simulink model "sim_quadrotor"  (R2015a)
settings: Solver=ode3  StartTime=0  StopTime=inf  FixedStep=quadEDT.sampletime  MaxStep=0.1  RelTol=1e-3
InitFcn:
  | % load parameters of the default quadrotor
  | disp('Quadrotor parameters loaded by InitFcn')
  | parameters_estimationcontrol %loads mdl_quadcopter, too!
  | 
  | % change to Simulation folder if in data folder
  | cd([matlabpath '/Simulation']);
undefined symbols (not defined in the file or in its folder): controlHelperParams, Discrete, estimParams, quad, quadEDT, Time
libraries: simulink x30, ctrlSharedLib x3, vrlib x1, commnoisgen2 x1, aerolibtransform2 x1
(part 2 of 2)

== system sim_quadrotor/Drone_Compensator/Estimator/EstimatorXYPosition/EstimatorXYPosition ==
  note: Switching from orientationControl to Position control reset the current world position estimate (happens when using no markers!)
  dxy_estimin : Inport
  orient_estimin : Inport  Port=2
  controlModePosVSOrient_flagin : Inport  Port=3
  dz_estimin : Inport  Port=4
  posVIS_datin : Inport  Port=5
  usePosVIS_flagin : Inport  Port=6
  Delay : Delay  DelayLength=1  InitialCondition=0
  KalmanFilter_posxy : ctrlSharedLib/Kalman Filter  TimeDomain=Discrete-Time  UseCurrentEstimator=on  ModelSource=Individual A, B, C, D matrices  ModelSourceVariable=ss(0.95,1,1,0,1)  A=eye(2)  B=quadEDT.sampletime*eye(2)  C=eye(2)  D=0  NumberOfStates=1  NumberOfInputs=1  NumberOfOutputs=1  InitialEstimateSource=Dialog  X0=[.1 0.0]  P0=10  UseK=off  UseGH=on  NumberOfProcessNoiseInputs=1  G=estimParams.pos.kfpos.G  TimeInvariantG=on  H=estimParams.pos.kfpos.H  TimeInvariantH=on  Q=estimParams.pos.kfpos.Q  TimeInvariantQ=on  R=estimParams.pos.kfpos.R  TimeInvariantR=on  N=estimParams.pos.kfpos.N  TimeInvariantN=on  AddInputPort=on  AddEnablePort=on  OutputEstimatedY=off  OutputP=off  Ts=-1
  Mux2 : Mux  Inputs=2
  OutlierHandling : Subsystem
  SelectXY : Selector  InputPortWidth=4  Indices=[1 2]
  SelectdXY : Selector  InputPortWidth=3  Indices=[1 2]
  SimplyIntegrateVelocity : DiscreteIntegrator  ExternalReset=rising  InitialConditionSetting=State (most efficient)  SampleTime=quadEDT.sampletime  LimitOutput=on  UpperSaturationLimit=estimParams.pos.veloIntegrator_max  LowerSaturationLimit=-estimParams.pos.veloIntegrator_max
  UseIPPosSwitch : Switch  Criteria=u2 > Threshold
  trafo_BodytoWorld_trans : MATLAB Function  TreatAsAtomicUnit=on
  XY_estimout : Outport
  wires:
  orient_estimin/1 -> trafo_BodytoWorld_trans/1(orientation), OutlierHandling/1(orient_estimin)
  dxy_estimin/1 -> Mux2/1
  SimplyIntegrateVelocity/1 -> UseIPPosSwitch/3
  dz_estimin/1 -> Mux2/2
  Mux2/1 -> trafo_BodytoWorld_trans/2(vector)
  trafo_BodytoWorld_trans/1(vel_world) -> SelectdXY/1
  SelectdXY/1 -> KalmanFilter_posxy/1, SimplyIntegrateVelocity/1
  posVIS_datin/1 -> SelectXY/1, OutlierHandling/2(posVIS_datin)
  KalmanFilter_posxy/1 -> Delay/1, UseIPPosSwitch/1
  controlModePosVSOrient_flagin/1 -> SimplyIntegrateVelocity/2
  UseIPPosSwitch/1 -> XY_estimout/1
  usePosVIS_flagin/1 -> UseIPPosSwitch/2
  SelectXY/1 -> KalmanFilter_posxy/2
  OutlierHandling/1(enable_flag) -> KalmanFilter_posxy/3
  Delay/1 -> OutlierHandling/3(pos_estim)

== system sim_quadrotor/SimulatorDrone/DroneRS_Sensorsystem/IMU_Pressure/ Noise ==
  states_datin : Inport
  Add : Sum
  Bus Creator : BusCreator  Inputs='X','Y','Z','yaw','pitch','roll','dx','dy','dz','p','q','r'
  Bus to Vector : BusToVector
  Demux1 : Demux  Outputs=12
  Gaussian Noise Generator : commnoisgen2/Gaussian Noise Generator  m=0  d=quadEDT.noiseStatesSensed_std.^2  s=41  Ts=quadEDT.sampletime  frameBased=off  sampPerFrame=1  orient=off  outDataType=double
  noiseWeights : Gain  Gain=quadEDT.noiseStatesSensed_weights
  states_noisy_datout : Outport
  wires:
  Bus Creator/1 -> states_noisy_datout/1
  Gaussian Noise Generator/1 -> noiseWeights/1
  Demux1/6 -> Bus Creator/6  "roll"
  Add/1 -> Demux1/1
  Demux1/8 -> Bus Creator/8  "dy"
  Demux1/10 -> Bus Creator/10  "p"
  Demux1/12 -> Bus Creator/12  "r"
  Demux1/2 -> Bus Creator/2  "Y"
  Bus to Vector/1 -> Add/1
  Demux1/3 -> Bus Creator/3  "Z"
  Demux1/7 -> Bus Creator/7  "dx"
  Demux1/9 -> Bus Creator/9  "dz"
  Demux1/4 -> Bus Creator/4  "yaw"
  Demux1/11 -> Bus Creator/11  "q"
  states_datin/1 -> Bus to Vector/1
  Demux1/5 -> Bus Creator/5  "pitch"
  Demux1/1 -> Bus Creator/1  "X"
  noiseWeights/1 -> Add/2

== system sim_quadrotor/Drone_Compensator/Estimator/EstimatorXYPosition/EstimatorVelocity/AccelerationHandling ==
  dxy_estimin : Inport
  orient_estimin : Inport  Port=2
  sensorIMU_datin : Inport  Port=3
  Z_estimin : Inport  Port=4
  Add : Sum  Inputs=-+
  Bus Selector1 : BusSelector  OutputSignals=ddx,ddy,ddz
  Deactivate Acceleration If OF is not used due to low altitude : simulink/Logic and Bit Operations/Compare To Constant  relop=<=  const=estimParams.pos.opticalFlow_Z_max  OutDataTypeStr=boolean
  Logical Operator : Logic  Operator=OR  AllPortsSameDT=off  OutDataTypeStr=boolean
  Mux6 : Mux  Inputs=3
  Product : Product  Inputs=3
  SelectPlanarddxy : Selector  InputPortWidth=3  Indices=[1 2]
  Selector : Selector  InputPortWidth=2
  Selector1 : Selector  InputPortWidth=2  Indices=2
  do not use acc if optical flow never available (Note OF@60Hz but ZOH to 200!) : simulink/Logic and Bit Operations/Compare To Constant  relop=~=  const=0  OutDataTypeStr=boolean
  do not use acc if optical flow never available (Note OF@60Hz but ZOH to 200!)1 : simulink/Logic and Bit Operations/Compare To Constant  relop=~=  const=0  OutDataTypeStr=boolean
  gainaccinput : Gain  Gain=estimParams.pos.accelerationInput_gain
  gravity : Constant  Value=[0 0 -quad.g]
  trafo_World2Body_trans : MATLAB Function  TreatAsAtomicUnit=on
  acceleration_world : Outport
  wires:
  orient_estimin/1 -> trafo_World2Body_trans/1(orientation)
  Bus Selector1/2 -> Mux6/2  "<ddy>"
  Mux6/1 -> Add/2
  sensorIMU_datin/1 -> Bus Selector1/1
  Bus Selector1/1 -> Mux6/1  "<ddx>"
  Bus Selector1/3 -> Mux6/3  "<ddz>"
  SelectPlanarddxy/1 -> gainaccinput/1
  gainaccinput/1 -> Product/2
  gravity/1 -> trafo_World2Body_trans/2(vector)
  trafo_World2Body_trans/1(y) -> Add/1
  Add/1 -> SelectPlanarddxy/1
  Z_estimin/1 -> Deactivate Acceleration If OF is not used due to low altitude/1
  Deactivate Acceleration If OF is not used due to low altitude/1 -> Product/3
  Product/1 -> acceleration_world/1
  dxy_estimin/1 -> Selector/1, Selector1/1
  Selector/1 -> do not use acc if optical flow never available (Note OF@60Hz but ZOH to 200!)/1
  Selector1/1 -> do not use acc if optical flow never available (Note OF@60Hz but ZOH to 200!)1/1
  Logical Operator/1 -> Product/1
  do not use acc if optical flow never available (Note OF@60Hz but ZOH to 200!)/1 -> Logical Operator/1
  do not use acc if optical flow never available (Note OF@60Hz but ZOH to 200!)1/1 -> Logical Operator/2

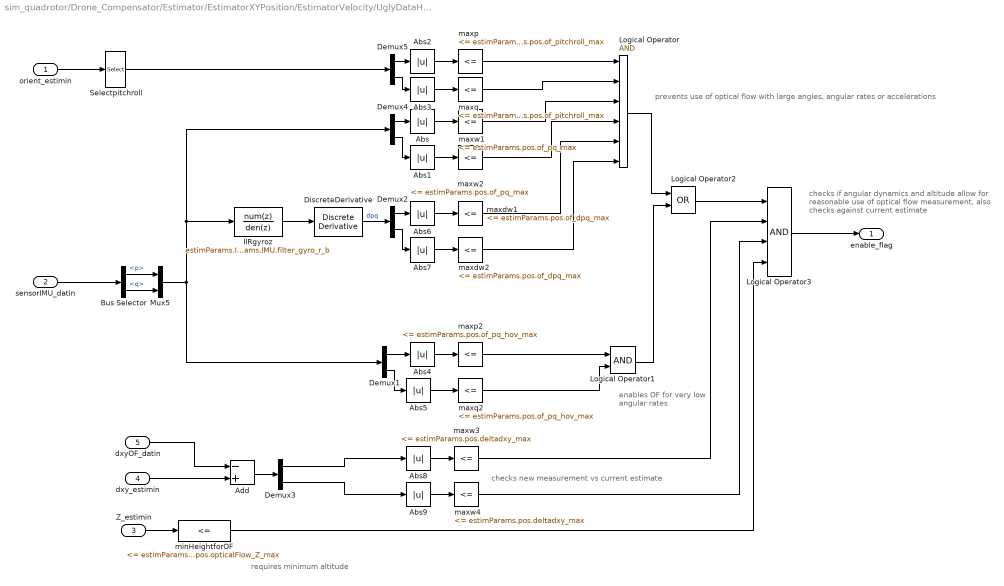
== system sim_quadrotor/Drone_Compensator/Estimator/EstimatorXYPosition/EstimatorVelocity/UglyDataHandling ==
  note: requires minimum altitude
  note: checks new measurement vs current estimate
  note: checks if angular dynamics and altitude allow for
      | reasonable use of optical flow measurement,
      | also checks against current estimate
  note: enables OF for very
      | low angular rates
  note: prevents use of optical flow with large angles, angular rates or accelerations
  orient_estimin : Inport
  sensorIMU_datin : Inport  Port=2
  Z_estimin : Inport  Port=3
  dxy_estimin : Inport  Port=4
  dxyOF_datin : Inport  Port=5
  Abs{,1..9} (10 alike) : Abs
  Add : Sum  Inputs=-+
  Bus Selector : BusSelector  OutputSignals=p,q
  Demux{1..5} (5 alike) : Demux  Outputs=2
  DiscreteDerivative : simulink/Discrete/Discrete Derivative  gainval=1.0  ICPrevScaledInput=0.0  InputProcessing=Inherited  OutMin=[]  OutMax=[]  OutDataType=fixdt(1, 16)  OutScaling=2^-10  DoSatur=off
  IIRgyroz : DiscreteFilter  Numerator=estimParams.IMU.filter_gyro_r_b  Denominator=estimParams.IMU.filter_gyro_r_b
  Logical Operator : Logic  Inputs=6  AllPortsSameDT=off  OutDataTypeStr=boolean
  Logical Operator1 : Logic  AllPortsSameDT=off  OutDataTypeStr=boolean
  Logical Operator2 : Logic  Operator=OR  AllPortsSameDT=off  OutDataTypeStr=boolean
  Logical Operator3 : Logic  Inputs=4  AllPortsSameDT=off  OutDataTypeStr=boolean
  Mux5 : Mux  Inputs=2
  Selectpitchroll : Selector  InputPortWidth=3  Indices=[2 3]
  maxdw1 : simulink/Logic and Bit Operations/Compare To Constant  relop=<=  const=estimParams.pos.of_dpq_max  OutDataTypeStr=boolean
  maxdw2 : simulink/Logic and Bit Operations/Compare To Constant  relop=<=  const=estimParams.pos.of_dpq_max  OutDataTypeStr=boolean
  maxp : simulink/Logic and Bit Operations/Compare To Constant  relop=<=  const=estimParams.pos.of_pitchroll_max  OutDataTypeStr=boolean
  maxp2 : simulink/Logic and Bit Operations/Compare To Constant  relop=<=  const=estimParams.pos.of_pq_hov_max  OutDataTypeStr=boolean
  maxq : simulink/Logic and Bit Operations/Compare To Constant  relop=<=  const=estimParams.pos.of_pitchroll_max  OutDataTypeStr=boolean
  maxq2 : simulink/Logic and Bit Operations/Compare To Constant  relop=<=  const=estimParams.pos.of_pq_hov_max  OutDataTypeStr=boolean
  maxw1 : simulink/Logic and Bit Operations/Compare To Constant  relop=<=  const=estimParams.pos.of_pq_max  OutDataTypeStr=boolean
  maxw2 : simulink/Logic and Bit Operations/Compare To Constant  relop=<=  const=estimParams.pos.of_pq_max  OutDataTypeStr=boolean
  maxw3 : simulink/Logic and Bit Operations/Compare To Constant  relop=<=  const=estimParams.pos.deltadxy_max  OutDataTypeStr=boolean
  maxw4 : simulink/Logic and Bit Operations/Compare To Constant  relop=<=  const=estimParams.pos.deltadxy_max  OutDataTypeStr=boolean
  minHeightforOF : simulink/Logic and Bit Operations/Compare To Constant  relop=<=  const=estimParams.pos.opticalFlow_Z_max  OutDataTypeStr=boolean
  enable_flag : Outport
  wires:
  maxp2/1 -> Logical Operator1/1
  Demux5/2 -> Abs3/1
  Demux5/1 -> Abs2/1
  maxq/1 -> Logical Operator/2
  maxdw2/1 -> Logical Operator/6
  maxdw1/1 -> Logical Operator/5
  orient_estimin/1 -> Selectpitchroll/1
  maxw2/1 -> Logical Operator/4
  maxp/1 -> Logical Operator/1
  Bus Selector/2 -> Mux5/2  "<q>"
  maxq2/1 -> Logical Operator1/2
  sensorIMU_datin/1 -> Bus Selector/1
  Selectpitchroll/1 -> Demux5/1
  Bus Selector/1 -> Mux5/1  "<p>"
  maxw1/1 -> Logical Operator/3
  Logical Operator/1 -> Logical Operator2/1
  Z_estimin/1 -> minHeightforOF/1
  Abs/1 -> maxw1/1
  Abs1/1 -> maxw2/1
  Demux4/1 -> Abs/1
  Demux4/2 -> Abs1/1
  Abs2/1 -> maxp/1
  Abs3/1 -> maxq/1
  Abs4/1 -> maxp2/1
  Abs5/1 -> maxq2/1
  Demux1/1 -> Abs4/1
  Demux1/2 -> Abs5/1
  Logical Operator1/1 -> Logical Operator2/2
  Abs6/1 -> maxdw1/1
  Abs7/1 -> maxdw2/1
  Demux2/1 -> Abs6/1
  Demux2/2 -> Abs7/1
  DiscreteDerivative/1 -> Demux2/1  "dpq"
  Logical Operator3/1 -> enable_flag/1
  Logical Operator2/1 -> Logical Operator3/1
  Abs8/1 -> maxw3/1
  Abs9/1 -> maxw4/1
  Add/1 -> Demux3/1
  dxy_estimin/1 -> Add/2
  Demux3/1 -> Abs8/1
  Demux3/2 -> Abs9/1
  dxyOF_datin/1 -> Add/1
  maxw3/1 -> Logical Operator3/2
  maxw4/1 -> Logical Operator3/3
  Mux5/1 -> Demux4/1, IIRgyroz/1, Demux1/1
  IIRgyroz/1 -> DiscreteDerivative/1
  minHeightforOF/1 -> Logical Operator3/4

== system sim_quadrotor/Drone_Compensator/Estimator/EstimatorXYPosition/EstimatorXYPosition/OutlierHandling ==
  orient_estimin : Inport
  posVIS_datin : Inport  Port=2
  pos_estim : Inport  Port=3
  Abs : Abs
  Abs1 : Abs
  Add1 : Sum  Inputs=+-
  Demux : Demux  Outputs=2
  Logical Operator3 : Logic  Inputs=4  AllPortsSameDT=off  OutDataTypeStr=boolean
  SelectX : Selector  InputPortWidth=4  Indices=[1]
  SelectXY : Selector  InputPortWidth=4  Indices=[1 2]
  Selector : Selector  InputPortWidth=3  Indices=[2 3]
  abs : MATLAB Function  TreatAsAtomicUnit=on
  checkifPosavailable : simulink/Logic and Bit Operations/Compare To Constant  relop=~=  const=-99  OutDataTypeStr=boolean
  maxp3 : simulink/Logic and Bit Operations/Compare To Constant  relop=<=  const=estimParams.pos.vis_orient_max  OutDataTypeStr=boolean
  maxq3 : simulink/Logic and Bit Operations/Compare To Constant  relop=<=  const=estimParams.pos.vis_orient_max  OutDataTypeStr=boolean
  planarjumpsVISPOS : simulink/Logic and Bit Operations/Compare To Constant  relop=<  const=estimParams.pos.vis_deltaXY_max  OutDataTypeStr=boolean
  enable_flag : Outport
  wires:
  posVIS_datin/1 -> SelectXY/1, SelectX/1
  SelectX/1 -> checkifPosavailable/1
  checkifPosavailable/1 -> Logical Operator3/1
  Logical Operator3/1 -> enable_flag/1
  maxp3/1 -> Logical Operator3/2
  maxq3/1 -> Logical Operator3/3
  SelectXY/1 -> Add1/1
  Add1/1 -> abs/1(vec)
  pos_estim/1 -> Add1/2
  abs/1(y) -> planarjumpsVISPOS/1
  planarjumpsVISPOS/1 -> Logical Operator3/4
  orient_estimin/1 -> Selector/1
  Selector/1 -> Demux/1
  Demux/1 -> Abs/1
  Demux/2 -> Abs1/1
  Abs/1 -> maxp3/1
  Abs1/1 -> maxq3/1

== matlab function sim_quadrotor/SimulatorDrone/Drone_Dynamics/MATLAB Function ==
  data: u input; y output; aomega2pwm input; bomega2pwm input; comega2pwm input
function y = fcn(u,aomega2pwm,bomega2pwm,comega2pwm)
y=sqrt((u-bomega2pwm)./aomega2pwm)+comega2pwm;

== matlab function sim_quadrotor/Drone_Compensator/ControllerPID/inverse rotation Function ==
  data: u input; y output
function y = fcn(u)
%inverse yaw-rotation
y = ([cos(u) sin(u); -sin(u) cos(u)]);

== matlab function sim_quadrotor/SimulatorDrone/DroneRS_Sensorsystem/IMU_Pressure/trafo_Body2World_trans ==
  data: orientation input; vector input; y output
function y = fcn(orientation,vector)

yaw     = orientation(1);
pitch   = orientation(2);
roll    = orientation(3);

R_Body2World =[ [ cos(pitch)*cos(yaw), cos(yaw)*sin(pitch)*sin(roll) - cos(roll)*sin(yaw), sin(roll)*sin(yaw) + cos(roll)*cos(yaw)*sin(pitch)];
[ cos(pitch)*sin(yaw), cos(roll)*cos(yaw) + sin(pitch)*sin(roll)*sin(yaw), cos(roll)*sin(pitch)*sin(yaw) - cos(yaw)*sin(roll)];
[         -sin(pitch),                               cos(pitch)*sin(roll),                              cos(pitch)*cos(roll)]];

y = R_Body2World*vector;

== matlab function sim_quadrotor/SimulatorDrone/DroneRS_Sensorsystem/IMU_Pressure/trafo_World2Body_trans ==
  data: orientation input; vector input; y output
function y = fcn(orientation,vector)

yaw     = orientation(1);
pitch   = orientation(2);
roll    = orientation(3);

R_World2Body = [[                                cos(pitch)*cos(yaw),                                cos(pitch)*sin(yaw),          -sin(pitch)];
                    [ cos(yaw)*sin(pitch)*sin(roll) - cos(roll)*sin(yaw), cos(roll)*cos(yaw) + sin(pitch)*sin(roll)*sin(yaw), cos(pitch)*sin(roll)];
                    [ sin(roll)*sin(yaw) + cos(roll)*cos(yaw)*sin(pitch), cos(roll)*sin(pitch)*sin(yaw) - cos(yaw)*sin(roll), cos(pitch)*cos(roll)]];

      
 y = R_World2Body*vector;

== matlab function sim_quadrotor/SimulatorDrone/Drone_Dynamics/Dynamics/MATLAB Function ==
  data: t input; x input; u input; dx output; quadverbose input; quadd input; quadh input; quadr input; quadtheta0 input; quadtheta1 input; quadgamma input; quadCt input; quadrho input; quadA input; quadCq input; quadg input; quadM input; quadJ input; motorTimeConstant input
%% drone derivatives
function dx = droneStateDerv(t,x,u, quadverbose,quadd,quadh,quadr,quadtheta0,quadtheta1,quadgamma,quadCt,quadrho,quadA,quadCq,quadg,quadM,quadJ,motorTimeConstant)
    %global a1s b1s
    %rebuilt quad.
quad.verbose=quadverbose;
quad.d=quadd;
quad.h=quadh;
quad.r=quadr;
quad.theta0=quadtheta0;
quad.theta1=quadtheta1;
quad.gamma=quadgamma;
quad.Ct=quadCt;
quad.rho=quadrho;
quad.A=quadA;
quad.Cq=quadCq;
quad.g=quadg;
quad.M=quadM;
quad.J=quadJ;
quadEDT.motorTimeConstant = motorTimeConstant;

%declarations/init
dz = zeros(3,1);
dv = zeros(3,1);
dn = zeros(3,1);
do = zeros(3,1);
dw = zeros(4,1);

a1s = zeros(4,1);
b1s = zeros(4,1);

T = zeros(3,4);
Q = zeros(3,4);
tau = zeros(3,4);

    %CONSTANTS
    %Cardinal Direction Indicies
    N = 1;                      %   N       'North'                             1x1
    E = 2;                      %   S       'South'                             1x1
    S = 3;                      %   E       'East'                              1x1
    W = 4;                      %   W       'West'                              1x1
    
    
    d=sqrt(2)/2*quad.d;
    
    D = zeros(3,4);
    
    D(:,1) = [ d;-d;quad.h];    %   Di      Rotor hub displacements             1x3
    D(:,2) = [ d; d;quad.h];
    D(:,3) = [-d; d;quad.h];
    D(:,4) = [-d;-d;quad.h]; 
    
    %Body-fixed frame references
    e1 = [1;0;0];               %   ei      Body fixed frame references         3x1
    e2 = [0;1;0];
    e3 = [0;0;1];
    
    %EXTRACT STATES FROM U
    w_ref = u(1:4);
    
    %EXTRACT STATES FROM X
    z = x(1:3);   % position in {W}
    n = x(4:6);   % RPY angles {W}
    v = x(7:9);   % velocity in {W}
    o = x(10:12); % angular velocity in {W} (body pqr? (F))
    w = x(13:16); % motor speed
    
    %PREPROCESS ROTATION AND WRONSKIAN MATRICIES
    phi = n(1);    % yaw
    the = n(2);    % pitch
    psi = n(3);    % roll

    if (abs(the)>pi/2) error('|pitch| greater than pi/2!'); end;
    if (abs(psi)>pi/2) error('|roll| greater than pi/2!'); end;
    %if (z(3)>0) error('z greater than 0 (under ground)!'); end;  

    
    % rotz(phi)*roty(the)*rotx(psi)
    R = [cos(the)*cos(phi) sin(psi)*sin(the)*cos(phi)-cos(psi)*sin(phi) cos(psi)*sin(the)*cos(phi)+sin(psi)*sin(phi);   %BBF > Inertial rotation matrix
         cos(the)*sin(phi) sin(psi)*sin(the)*sin(phi)+cos(psi)*cos(phi) cos(psi)*sin(the)*sin(phi)-sin(psi)*cos(phi);
         -sin(the)         sin(psi)*cos(the)                            cos(psi)*cos(the)];
    
    
    %Manual Construction
    %     Q3 = [cos(phi) -sin(phi) 0;sin(phi) cos(phi) 0;0 0 1];   % RZ %Rotation mappings
    %     Q2 = [cos(the) 0 sin(the);0 1 0;-sin(the) 0 cos(the)];   % RY
    %     Q1 = [1 0 0;0 cos(psi) -sin(psi);0 sin(psi) cos(psi)];   % RX
    %     R = Q3*Q2*Q1    %Rotation matrix
    %
    %    RZ * RY * RX
    iW = [0        sin(psi)          cos(psi);             %inverted Wronskian (body rates p-q-r to euler rates yaw pitch roll)
          0        cos(psi)*cos(the) -sin(psi)*cos(the);
          cos(the) sin(psi)*sin(the) cos(psi)*sin(the)] / cos(the);
    
    %ROTOR MODEL
    for i=[N E S W] %for each rotor
        %Relative motion
        
        Vr = cross(o,D(:,i)) + inv(R)*v;
        mu = sqrt(sum(Vr(1:2).^2)) / (abs(w(i))*quad.r);  %Magnitude of mu, planar components
        lc = Vr(3) / (abs(w(i))*quad.r);                  %Non-dimensionalised normal inflow
        li = mu;                                          %Non-dimensionalised induced velocity approximation
        alphas = atan2(lc,mu);
        j = atan2(Vr(2),Vr(1));                           %Sideslip azimuth relative to e1 (zero over nose)
        J = [cos(j) -sin(j);
            sin(j) cos(j)];                               %BBF > mu sideslip rotation matrix
        
        %Flapping
        beta = [((8/3*quad.theta0 + 2*quad.theta1)*mu - 2*(lc)*mu)/(1-mu^2/2); %Longitudinal flapping
            0;];                                          %sign(w) * (4/3)*((Ct/sigma)*(2*mu*gamma/3/a)/(1+3*e/2/r) + li)/(1+mu^2/2)]; %Lattitudinal flapping (note sign)
        beta = J'*beta;                                   %Rotate the beta flapping angles to longitudinal and lateral coordinates.
        a1s(i) = beta(1) - 16/quad.gamma/abs(w(i)) * o(2);
        b1s(i) = beta(2) - 16/quad.gamma/abs(w(i)) * o(1);
        
        %Forces and torques
        T(:,i) = quad.Ct*quad.rho*quad.A*quad.r^2*w(i)^2 * [-cos(b1s(i))*sin(a1s(i)); sin(b1s(i));-cos(a1s(i))*cos(b1s(i))];   %Rotor thrust, linearised angle approximations
        Q(:,i) = -quad.Cq*quad.rho*quad.A*quad.r^3*w(i)*abs(w(i)) * e3;     %Rotor drag torque - note that this preserves w(i) direction sign
        %tau(:,i) = cross(T(:,i),D(:,i));                %Torque due to rotor thrust
        tau(:,i) = cross(D(:,i),T(:,i));                 %changed sign (F)
    end
    
    %RIGID BODY DYNAMIC MODEL
    dz = v;
    dn = iW*o;
    
    dv = (quad.g*e3 + R*(1/quad.M)*sum(T,2));
    do = inv(quad.J)*(-cross(o,quad.J*o) + sum(tau,2) + sum(Q,2)); %row sum of torques
    
    dw = 1/quadEDT.motorTimeConstant*(w_ref-w);
    
    dx = [dz;dn;dv;do;dw];                                           %This is the state derivative vector
    
    
    
end % End of mdlDerivatives.

== matlab function sim_quadrotor/Drone_Compensator/Estimator/EstimatorXYPosition/EstimatorVelocity/AccelerationHandling/trafo_World2Body_trans ==
  data: orientation input; vector input; y output
function y = fcn(orientation,vector)

yaw     = orientation(1);
pitch   = orientation(2);
roll    = orientation(3);

R_World2Body = [[                                cos(pitch)*cos(yaw),                                cos(pitch)*sin(yaw),          -sin(pitch)];
                    [ cos(yaw)*sin(pitch)*sin(roll) - cos(roll)*sin(yaw), cos(roll)*cos(yaw) + sin(pitch)*sin(roll)*sin(yaw), cos(pitch)*sin(roll)];
                    [ sin(roll)*sin(yaw) + cos(roll)*cos(yaw)*sin(pitch), cos(roll)*sin(pitch)*sin(yaw) - cos(yaw)*sin(roll), cos(pitch)*cos(roll)]];

y = R_World2Body*vector;

== matlab function sim_quadrotor/SimulatorDrone/Drone_Dynamics/Dynamics/statetoout ==
  data: t input; x input; sys output; quadverbose input; quadd input; quadh input; quadr input; quadtheta0 input; quadtheta1 input; quadgamma input; quadCt input; quadrho input; quadA input; quadCq input; quadg input; quadM input; quadJ input
%==============================================================
% mdlOutputs
% Calculate the output vector for this timestep
%==============================================================
%
function sys = droneOutputs(t,x, quadverbose,quadd,quadh,quadr,quadtheta0,quadtheta1,quadgamma,quadCt,quadrho,quadA,quadCq,quadg,quadM,quadJ)

%rebuilt quad.
quad.verbose=quadverbose;
quad.d=quadd;
quad.h=quadh;
quad.r=quadr;
quad.theta0=quadtheta0;
quad.theta1=quadtheta1;
quad.gamma=quadgamma;
quad.Ct=quadCt;
quad.rho=quadrho;
quad.A=quadA;
quad.Cq=quadCq;
quad.g=quadg;
quad.M=quadM;
quad.J=quadJ;

    %CRASH DETECTION
%     if x(3)>0
%         x(3) = 0;
%         if x(6) > 0
%             x(6) = 0;
%         end
%     end
    %if (x(3)>0)&(crash)
    %    error('CRASH!')
    %end
    
    %TELEMETRY
    if quad.verbose
        %disp(sprintf('%0.3f\t',t,x))
    end
    
    % compute output vector as a function of state vector
    %   z      Position                         3x1   (x,y,z)
    %   v      Velocity                         3x1   (xd,yd,zd)
    %   n      Attitude                         3x1   (Y,P,R)
    %   o      Angular velocity                 3x1   (Yd,Pd,Rd)
    
    n = x(4:6);   % RPY angles
    phi = n(1);    % yaw
    the = n(2);    % pitch
    psi = n(3);    % roll
    
    
    % rotz(phi)*roty(the)*rotx(psi)
    R = [cos(the)*cos(phi) sin(psi)*sin(the)*cos(phi)-cos(psi)*sin(phi) cos(psi)*sin(the)*cos(phi)+sin(psi)*sin(phi);   %BBF > Inertial rotation matrix
         cos(the)*sin(phi) sin(psi)*sin(the)*sin(phi)+cos(psi)*cos(phi) cos(psi)*sin(the)*sin(phi)-sin(psi)*cos(phi);
         -sin(the)         sin(psi)*cos(the)                            cos(psi)*cos(the)];
    
    iW = [0        sin(psi)          cos(psi);             %inverted Wronskian
          0        cos(psi)*cos(the) -sin(psi)*cos(the);
          cos(the) sin(psi)*sin(the) cos(psi)*sin(the)] / cos(the);
    
    % return velocity in the body frame
    sys = [ x(1:6);             %output global pos and euler angles
            inv(R)*x(7:9);      %translational velocity mapped to body frame -> i.e. output v in bodyframe! (F)
            x(10:12);%iW*x(10:12)];    % RPY rates mapped to body frame ->     i.e. : this outputed euler rates!, now in bodyrates pqr (F)
            x(13:16)]; %motor speed
    %sys = [x(1:6); iW*x(7:9);  iW*x(10:12)];
    %sys = x;
end
% End of mdlOutputs.

== matlab function sim_quadrotor/Drone_Compensator/Estimator/EstimatorXYPosition/EstimatorXYPosition/trafo_BodytoWorld_trans ==
  data: orientation input; vector input; vel_world output
function vel_world = fcn(orientation,vector)
yaw   = orientation(1);
pitch = orientation(2);
roll  = orientation(3);

R_BodytoWorld = [cos(pitch)*cos(yaw) sin(roll)*sin(pitch)*cos(yaw)-cos(roll)*sin(yaw) cos(roll)*sin(pitch)*cos(yaw)+sin(roll)*sin(yaw);   %BBF > Inertial rotation matrix
  cos(pitch)*sin(yaw) sin(roll)*sin(pitch)*sin(yaw)+cos(roll)*cos(yaw) cos(roll)*sin(pitch)*sin(yaw)-sin(roll)*cos(yaw);
  -sin(pitch)         sin(roll)*cos(pitch)                            cos(roll)*cos(pitch)];

vel_world = R_BodytoWorld*vector;

== matlab function sim_quadrotor/Drone_Compensator/Estimator/EstimatorAltitude/trafo_BodytoWorld_trans ==
  data: orientation input; vector input; acc_world output
function acc_world = fcn(orientation,vector)
yaw     = orientation(1);
pitch   = orientation(2);
roll    = orientation(3);

R_BodytoWorld = [cos(pitch)*cos(yaw) sin(roll)*sin(pitch)*cos(yaw)-cos(roll)*sin(yaw) cos(roll)*sin(pitch)*cos(yaw)+sin(roll)*sin(yaw);   %BBF > Inertial rotation matrix
  cos(pitch)*sin(yaw) sin(roll)*sin(pitch)*sin(yaw)+cos(roll)*cos(yaw) cos(roll)*sin(pitch)*sin(yaw)-sin(roll)*cos(yaw);
  -sin(pitch)         sin(roll)*cos(pitch)                            cos(roll)*cos(pitch)];

acc_world = R_BodytoWorld*vector;

== matlab function sim_quadrotor/Drone_Compensator/Estimator/EstimatorAltitude/trafo_WorldToBody_trans ==
  data: orientation input; vector input; acc_RS output
function acc_RS = fcn(orientation,vector)
yaw     = orientation(1);
pitch   = orientation(2);
roll    = orientation(3);


R_World2Body = [[                                cos(pitch)*cos(yaw),                                cos(pitch)*sin(yaw),          -sin(pitch)];
                    [ cos(yaw)*sin(pitch)*sin(roll) - cos(roll)*sin(yaw), cos(roll)*cos(yaw) + sin(pitch)*sin(roll)*sin(yaw), cos(pitch)*sin(roll)];
                    [ sin(roll)*sin(yaw) + cos(roll)*cos(yaw)*sin(pitch), cos(roll)*sin(pitch)*sin(yaw) - cos(yaw)*sin(roll), cos(pitch)*cos(roll)]];

acc_RS = R_World2Body*vector;

== matlab function sim_quadrotor/Drone_Compensator/Estimator/EstimatorOrientation ==
  data: sensorIMU_datin input; yawVIS_datin input; validVIS_flagin input; g input; orient_estimout output; dt input; dorient_estimout output; deuler_datout output; imuAbs_datout output
function [orient_estimout, dorient_estimout,deuler_datout,imuAbs_datout]  = fcn(sensorIMU_datin, yawVIS_datin, validVIS_flagin, g, dt)
persistent yaw_cur pitch_cur roll_cur

p = sensorIMU_datin(4);
q = sensorIMU_datin(5);
r = sensorIMU_datin(6);

if isempty(yaw_cur)
   yaw_cur = 0;
end
if isempty(pitch_cur)
   pitch_cur = 0;
end
if isempty(roll_cur)
   roll_cur = 0;
end

[yaw,pitch,roll,deuler_datout,imuAbs_datout]= complimentaryfilter(yaw_cur, pitch_cur, roll_cur, g, dt,sensorIMU_datin, yawVIS_datin,validVIS_flagin);

yaw_cur     = yaw;
pitch_cur   = pitch;
roll_cur    = roll;

orient_estimout     = [yaw,pitch,roll]';
dorient_estimout    = [p,q,r]';

== matlab function sim_quadrotor/Drone_Compensator/Estimator/EstimatorXYPosition/EstimatorXYPosition/OutlierHandling/abs ==
  data: vec input; y output
function y = fcn(vec)
y = norm(vec,2);

== matlab function sim_quadrotor/3D-VR-Animation/Euler angle rotations ==
  data: rot_phi output; rot_theta output; O input; rot_psi output
function [rot_phi,rot_theta,rot_psi] = fcn(O)
% @Erlend Solbakk Harbitz
% Calculate three axis of rotation with corresponding angles. This is the
% Euler angle approach as eigenvectors of the rotation matrix didn't
% work (returned complex eigenvectors)...

% In each of the three outputs the first three elements give the vector of
% rotation and the forth element gives the magnitude (angle)

psi   = O(1);
theta = O(2);
phi   = O(3);

rot_psi   = [0;0;1;psi];
rot_theta = [-sin(psi);cos(psi);0;theta];
rot_phi   = [cos(theta)*cos(psi);sin(psi);-sin(theta)*sin(psi);phi];

end
